simulink model "Q6_a"  (R2017a)
settings: Solver=FixedStepAuto  StartTime=0.0  StopTime=10  FixedStep=0.01  RelTol=0.00001
model workspace (MAT data in the model file):
  Kp_1 = 10000
  Kp_2 = 10000
  Kv_1 = 200
  Kv_2 = 200
  a_1 = 1
  a_2 = 1
  g = 9.8
  m_1 = 1
  m_2 = 1
  theta_d_dot = 0.314159265359
  theta_d_double_dot = 0.314159265359
undefined symbols (not defined in the file): DiscIntNeverNeededParam
libraries: simulink x3
settings Model: Creator=Omer  LastModifiedBy=Omer
settings ModelReferenceCC: ModelReferenceMinAlgLoopOccurrences=on

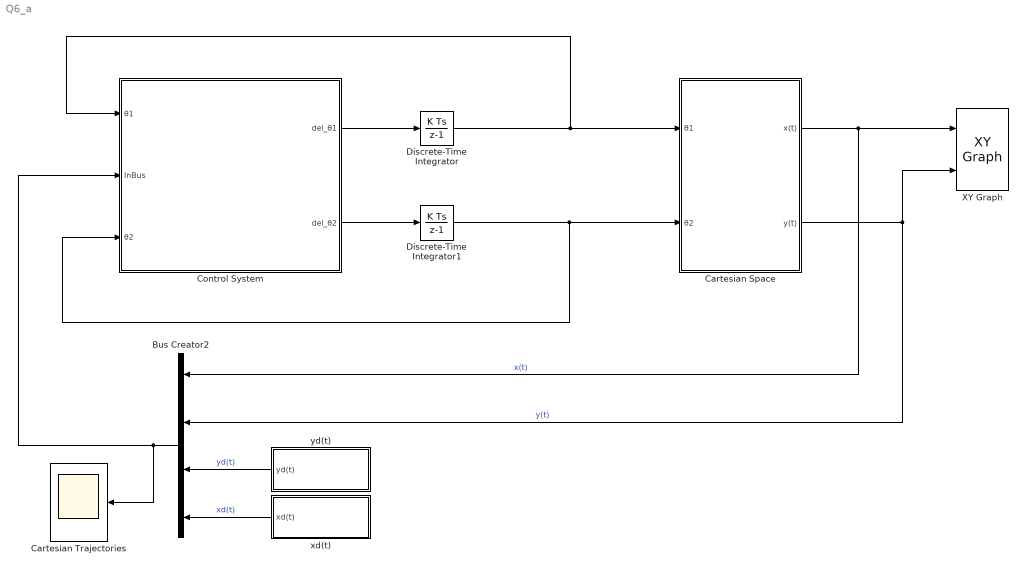
== system Q6_a ==
  Bus Creator2 : BusCreator  Inputs=4
  "Cartesian Space " : Subsystem  TreatAsAtomicUnit=on
  Cartesian Trajectories : Scope
  Control System : Subsystem  TreatAsAtomicUnit=on
  Discrete-Time Integrator : DiscreteIntegrator  gainval=1  InitialConditionSetting=State (most efficient)  SampleTime=-1  ICPrevOutput=DiscIntNeverNeededParam  ICPrevScaledInput=DiscIntNeverNeededParam
  Discrete-Time Integrator1 : DiscreteIntegrator  gainval=1  InitialConditionSetting=State (most efficient)  SampleTime=-1  ICPrevOutput=DiscIntNeverNeededParam  ICPrevScaledInput=DiscIntNeverNeededParam
  XY Graph : simulink/Sinks/XY Graph  xmin=-3  xmax=3  ymin=-3  ymax=3  st=-1
  xd(t) : Subsystem  TreatAsAtomicUnit=on
  yd(t) : Subsystem  TreatAsAtomicUnit=on
  wires:
  Control System/1(del_θ1) -> Discrete-Time Integrator/1
  "Cartesian Space "/1(x(t)) -> Bus Creator2/1, XY Graph/1  "x(t)"
  "Cartesian Space "/2(y(t)) -> XY Graph/2, Bus Creator2/2  "y(t)"
  Bus Creator2/1 -> Cartesian Trajectories/1, Control System/2(InBus)
  xd(t)/1(xd(t)) -> Bus Creator2/4  "xd(t)"
  yd(t)/1(yd(t)) -> Bus Creator2/3  "yd(t)"
  Discrete-Time Integrator/1 -> Control System/1(θ1), "Cartesian Space "/1(θ1)
  Discrete-Time Integrator1/1 -> "Cartesian Space "/2(θ2), Control System/3(θ2)
  Control System/2(del_θ2) -> Discrete-Time Integrator1/1

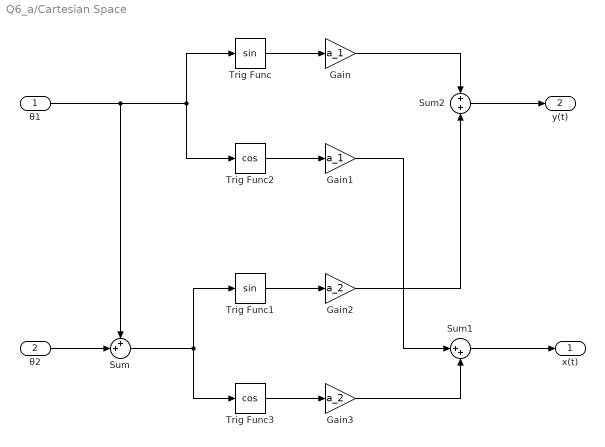
== system Q6_a/Cartesian Space  ==
  θ1 : Inport
  θ2 : Inport  Port=2
  Gain : Gain  Gain=a_1
  Gain1 : Gain  Gain=a_1
  Gain2 : Gain  Gain=a_2
  Gain3 : Gain  Gain=a_2
  Sum : Sum  Inputs=++|
  Sum1 : Sum  Inputs=|++
  Sum2 : Sum  Inputs=+|+
  Trig Func : Trigonometry
  Trig Func1 : Trigonometry
  Trig Func2 : Trigonometry  Operator=cos
  Trig Func3 : Trigonometry  Operator=cos
  x(t) : Outport
  y(t) : Outport  Port=2
  wires:
  θ1/1 -> Trig Func2/1, Trig Func/1, Sum/1
  θ2/1 -> Sum/2
  Sum/1 -> Trig Func3/1, Trig Func1/1
  Sum2/1 -> y(t)/1
  Sum1/1 -> x(t)/1
  Trig Func/1 -> Gain/1
  Gain/1 -> Sum2/1
  Trig Func2/1 -> Gain1/1
  Gain1/1 -> Sum1/1
  Trig Func1/1 -> Gain2/1
  Gain2/1 -> Sum2/2
  Trig Func3/1 -> Gain3/1
  Gain3/1 -> Sum1/2

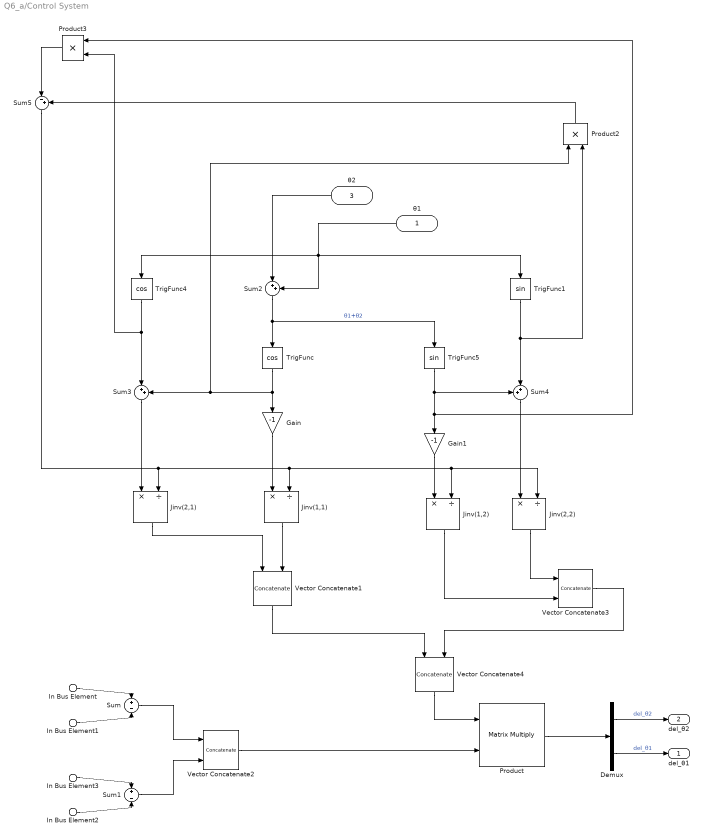
== system Q6_a/Control System ==
  θ1 : Inport
  In Bus Element1 : Inport  Port=2  PortName=InBus  Element=x(t)
  In Bus Element2 : Inport  Port=2  PortName=InBus  Element=y(t)
  In Bus Element : Inport  Port=2  PortName=InBus  Element=xd(t)
  In Bus Element3 : Inport  Port=2  PortName=InBus  Element=yd(t)
  θ2 : Inport  Port=3
  Demux : Demux  Outputs=2
  Gain : Gain  Gain=-1
  Gain1 : Gain  Gain=-1
  Jinv(1,1) : Product  Inputs=*/
  Jinv(1,2) : Product  Inputs=*/
  Jinv(2,1) : Product  Inputs=*/
  Jinv(2,2) : Product  Inputs=*/
  Product : Product  Multiplication=Matrix(*)
  Product2 : Product
  Product3 : Product
  Sum : Sum  Inputs=+|-
  Sum1 : Sum  Inputs=+|-
  Sum2 : Sum  Inputs=|++
  Sum3 : Sum  Inputs=|++
  Sum4 : Sum  Inputs=++|
  Sum5 : Sum  Inputs=|-+
  TrigFunc : Trigonometry  Operator=cos
  TrigFunc1 : Trigonometry
  TrigFunc4 : Trigonometry  Operator=cos
  TrigFunc5 : Trigonometry
  Vector Concatenate1 : Concatenate  Mode=Multidimensional array
  Vector Concatenate2 : Concatenate  Mode=Multidimensional array
  Vector Concatenate3 : Concatenate  Mode=Multidimensional array
  Vector Concatenate4 : Concatenate  Mode=Multidimensional array  ConcatenateDimension=2
  del_θ1 : Outport
  del_θ2 : Outport  Port=2
  wires:
  In Bus Element3/1 -> Sum1/1
  In Bus Element2/1 -> Sum1/2
  In Bus Element/1 -> Sum/1
  In Bus Element1/1 -> Sum/2
  Sum/1 -> Vector Concatenate2/1
  Sum1/1 -> Vector Concatenate2/2
  Sum2/1 -> TrigFunc/1, TrigFunc5/1  "θ1+θ2"
  TrigFunc4/1 -> Product3/2, Sum3/1
  TrigFunc/1 -> Product2/1, Sum3/2, Gain/1
  TrigFunc5/1 -> Product3/1, Gain1/1, Sum4/1
  TrigFunc1/1 -> Product2/2, Sum4/2
  Product2/1 -> Sum5/2
  Sum5/1 -> Jinv(2,2)/2, Jinv(1,2)/2, Jinv(1,1)/2, Jinv(2,1)/2
  Sum3/1 -> Jinv(2,1)/1
  Gain/1 -> Jinv(1,1)/1
  Sum4/1 -> Jinv(2,2)/1
  Product/1 -> Demux/1
  θ1/1 -> Sum2/2, TrigFunc1/1, TrigFunc4/1
  θ2/1 -> Sum2/1
  Demux/2 -> del_θ1/1  "del_θ1"
  Demux/1 -> del_θ2/1  "del_θ2"
  Vector Concatenate4/1 -> Product/1
  Vector Concatenate2/1 -> Product/2
  Jinv(1,1)/1 -> Vector Concatenate1/2
  Jinv(2,1)/1 -> Vector Concatenate1/1
  Product3/1 -> Sum5/1
  Vector Concatenate1/1 -> Vector Concatenate4/1
  Vector Concatenate3/1 -> Vector Concatenate4/2
  Jinv(2,2)/1 -> Vector Concatenate3/1
  Gain1/1 -> Jinv(1,2)/1
  Jinv(1,2)/1 -> Vector Concatenate3/2

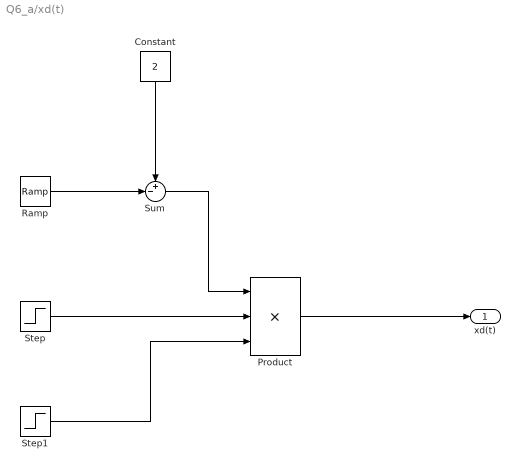
== system Q6_a/xd(t) ==
  Constant : Constant  Value=2
  Product : Product  Inputs=3
  Ramp : simulink/Sources/Ramp  slope=1  start=0  X0=0
  Step : Step  Time=0  SampleTime=0
  Step1 : Step  Time=2  Before=1  After=0  SampleTime=0
  Sum : Sum  Inputs=+-|
  xd(t) : Outport
  wires:
  Product/1 -> xd(t)/1
  Step/1 -> Product/2
  Step1/1 -> Product/3
  Constant/1 -> Sum/1
  Ramp/1 -> Sum/2
  Sum/1 -> Product/1

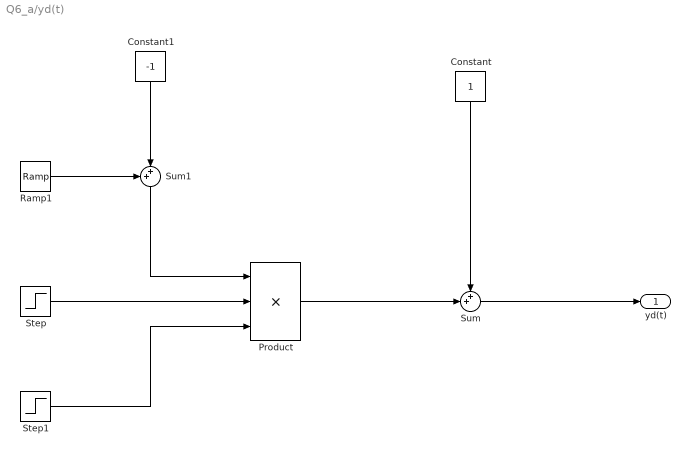
== system Q6_a/yd(t) ==
  Constant : Constant
  Constant1 : Constant  Value=-1
  Product : Product  Inputs=3
  Ramp1 : simulink/Sources/Ramp  slope=0.5  start=0  X0=0
  Step : Step  Time=0  SampleTime=0
  Step1 : Step  Time=2  Before=1  After=0  SampleTime=0
  Sum : Sum  Inputs=++|
  Sum1 : Sum  Inputs=++|
  yd(t) : Outport
  wires:
  Step1/1 -> Product/3
  Step/1 -> Product/2
  Sum/1 -> yd(t)/1
  Constant/1 -> Sum/1
  Product/1 -> Sum/2
  Ramp1/1 -> Sum1/1
  Constant1/1 -> Sum1/2
  Sum1/1 -> Product/1
